simulink model "Insulin_SubsystemReal"  (R2019a)
settings: Solver=VariableStepAuto  StartTime=0.0  StopTime=4  RelTol=1e-3
undefined symbols (not defined in the file): Q_i_P, V_i_PF
settings Model: Creator=cgonterman  LastModifiedBy=rache
settings DataIOCC: ReturnWorkspaceOutputs=off
settings DebuggingCC: PregeneratedLibrarySubsystemCodeDiagnostic=none  ArithmeticOperatorsInVariantConditions=warning
settings ModelReferenceCC: ModelReferenceMinAlgLoopOccurrences=on
settings SFSimCC: SimUseLocalCustomCode=off
settings RTWCC: RTWUseLocalCustomCode=off

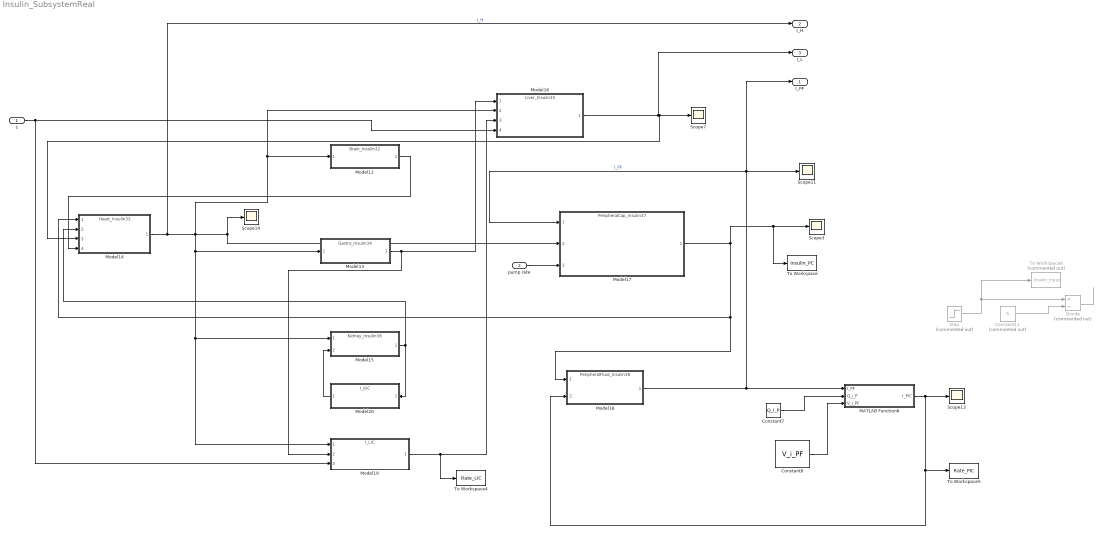
== system Insulin_SubsystemReal ==
  s : Inport  OutMin=0
  pump rate : Inport  Port=2
  Constant11 : Constant  Commented=on  Value=5
  Constant7 : Constant  Value=Q_i_P
  Constant8 : Constant  Value=V_i_PF
  Divide : Product  Commented=on  Inputs=*/
  MATLAB Function6 : MATLAB Function  TreatAsAtomicUnit=on
  Model12 : ModelReference  ModelNameDialog=Brain_Insulin32  SimulationMode=Normal  ModelReferenceVersion=1.3
  Model13 : ModelReference  ModelNameDialog=Gastro_Insulin34  SimulationMode=Normal  ModelReferenceVersion=1.3
  Model14 : ModelReference  ModelNameDialog=Heart_Insulin33  SimulationMode=Normal  ModelReferenceVersion=1.8
  Model15 : ModelReference  ModelNameDialog=Kidney_Insulin36  SimulationMode=Normal  ModelReferenceVersion=1.7
  Model16 : ModelReference  ModelNameDialog=Liver_Insulin35  SimulationMode=Normal  ModelReferenceVersion=1.7
  Model17 : ModelReference  ModelNameDialog=PeripheralCap_Insulin37  SimulationMode=Normal  ModelReferenceVersion=1.9
  Model18 : ModelReference  ModelNameDialog=PeripheralFluid_Insulin38  SimulationMode=Normal  ModelReferenceVersion=1.4
  Model19 : ModelReference  ModelNameDialog=r_LIC  SimulationMode=Normal  ModelReferenceVersion=1.2
  Model20 : ModelReference  ModelNameDialog=r_KIC  SimulationMode=Normal  ModelReferenceVersion=1.1
  Scope{3,7,11,13..14} (5 alike) : Scope
  Step : Step  Commented=on  Time=800  After=8  SampleTime=0
  To Workspace : ToWorkspace  VariableName=Insulin_PC  SaveFormat=Structure With Time  SampleTime=-1
  To Workspace4 : ToWorkspace  VariableName=Rate_LIC  SaveFormat=Structure With Time  SampleTime=-1
  To Workspace5 : ToWorkspace  VariableName=Rate_PIC  SaveFormat=Structure With Time  SampleTime=-1
  To Workspace6 : ToWorkspace  Commented=on  VariableName=Insulin_Input  SaveFormat=Structure With Time  SampleTime=-1
  I_PF : Outport  OutMin=0
  I_H : Outport  Port=2  OutMin=0
  I_L : Outport  Port=3
  wires:
  Model19/1 -> To Workspace4/1, Model16/3
  Model15/1 -> Model14/2, Model20/1
  Model18/1 -> Model17/1, I_PF/1, Scope11/1, MATLAB Function6/1(I_PF)  "I_PF"
  Divide/1 -> ?
  Step/1 -> Divide/1, To Workspace6/1
  Model13/1 -> Model19/2, Model16/1
  Constant8/1 -> MATLAB Function6/3(V_i_PF)
  MATLAB Function6/1(r_PIC) -> Scope13/1, To Workspace5/1, Model18/2
  Model12/1 -> Model14/4
  Constant7/1 -> MATLAB Function6/2(Q_i_P)
  Model14/1 -> I_H/1, Model13/1, Model15/1, Model19/1, Model16/2, Model12/1, Scope14/1, Model17/2  "I_H"
  Model17/1 -> To Workspace/1, Scope3/1, Model18/1, Model14/1
  Model16/1 -> I_L/1, Model14/3, Scope7/1
  Constant11/1 -> Divide/2
  Model20/1 -> Model15/2
  s/1 -> Model19/3, Model16/4
  pump rate/1 -> Model17/3

== matlab function Insulin_SubsystemReal/MATLAB Function6 ==
  data: I_PF input; r_PIC output; Q_i_P input; V_i_PF input
function r_PIC = fcn(I_PF, Q_i_P, V_i_PF)
r_PIC=I_PF/(((1-0.15)/(0.15*Q_i_P))-(20/V_i_PF));
